simulink model "SistemaCAS_v32"  (R2014a)
settings: Solver=ode45  StartTime=0.0  StopTime=100.0  RelTol=1e-3
libraries: simulink x1, dspsrcs4 x1
settings Model: Creator=andre  LastModifiedBy=andre

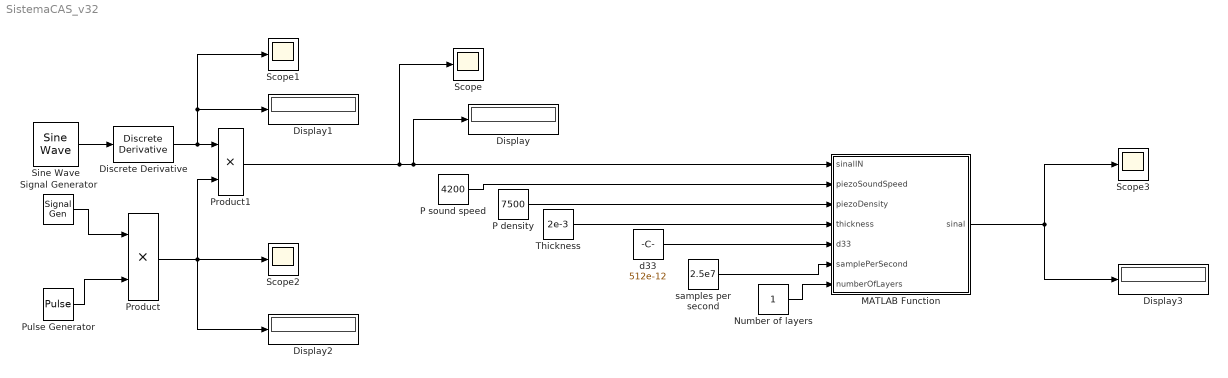
== system SistemaCAS_v32 ==
  Discrete Derivative : simulink/Discrete/Discrete Derivative  gainval=1.0  ICPrevScaledInput=0.0  InputProcessing=Inherited  OutMin=[]  OutMax=[]  OutDataType=fixdt(1, 16)  OutScaling=2^-10  DoSatur=off
  Display{,1..3} (4 alike) : Display
  MATLAB Function : MATLAB Function  TreatAsAtomicUnit=on
  Number of layers : Constant
  P density : Constant  Value=7500
  P sound speed : Constant  Value=4200
  Product : Product
  Product1 : Product
  Pulse Generator : DiscretePulseGenerator  Period=10  PulseWidth=5
  Scope{,1..3} (4 alike) : Scope
      Scope2 settings: SaveName=ScopeData2
      Scope3 settings: SaveName=ScopeData3
  Signal Generator : SignalGenerator  Amplitude=2  Frequency=5  Units=rad/sec
  Sine Wave : dspsrcs4/Sine Wave  Amplitude=10  Frequency=5  Phase=0  SampleMode=Discrete  OutComplex=Real  CompMethod=Trigonometric fcn  TableSize=Speed  SampleTime=1/1000  SamplesPerFrame=1  ResetState=Restart at time zero  dataType=double  wordLen=16  udDataType=sfix(16)  fracBitsMode=Best precision  numFracBits=15  OutDataTypeStr=double  LastOutDataTypeStr=double
  Thickness : Constant  Value=2e-3
  d33 : Constant  Value=512e-12
  samples per second : Constant  Value=2.5e7
  wires:
  Discrete Derivative/1 -> Display1/1, Scope1/1, Product1/1
  Signal Generator/1 -> Product/1
  Product/1 -> Display2/1, Scope2/1, Product1/2
  Sine Wave/1 -> Discrete Derivative/1
  Pulse Generator/1 -> Product/2
  d33/1 -> MATLAB Function/5(d33)
  samples per second/1 -> MATLAB Function/6(samplePerSecond)
  Number of layers/1 -> MATLAB Function/7(numberOfLayers)
  Product1/1 -> Display/1, MATLAB Function/1(sinalIN), Scope/1
  P sound speed/1 -> MATLAB Function/2(piezoSoundSpeed)
  P density/1 -> MATLAB Function/3(piezoDensity)
  Thickness/1 -> MATLAB Function/4(thickness)
  MATLAB Function/1(sinal) -> Display3/1, Scope3/1

== matlab function SistemaCAS_v32/MATLAB Function ==
  data: sinalIN input; sinal output; piezoSoundSpeed input; piezoDensity input; thickness input; d33 input; samplePerSecond input; numberOfLayers input
function sinal = projetor(sinalIN, piezoSoundSpeed, piezoDensity, thickness, d33, samplePerSecond, numberOfLayers)

sinal=sinalIN;
